simulink model "dlqr_reg_lin_model"  (R2017a)
settings: Solver=ode5  StartTime=0.0  StopTime=7  FixedStep=0.0056  RelTol=1e-3
values from neighbouring files (symbols this model uses):
  A = sys_ss.A    [dlqr_reg.m]
  B = sys_ss.B(:,1)    [dlqr_reg.m]
  C = sys_ss.C    [dlqr_reg.m]
  D = sys_ss.D(1)    [dlqr_reg.m]
undefined symbols (not defined in the file or in its folder): DiscIntNeverNeededParam, K1
libraries: cstblocks x1
settings Model: Creator=user  LastModifiedBy=user

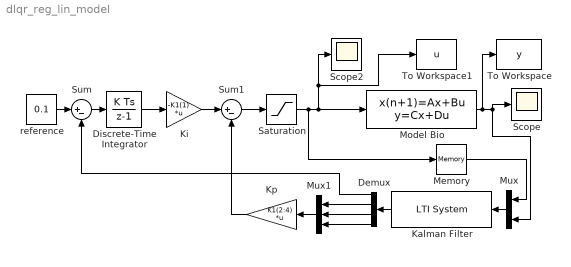
== system dlqr_reg_lin_model ==
  Demux : Demux
  Discrete-Time Integrator : DiscreteIntegrator  InitialConditionSetting=State (most efficient)  SampleTime=-1  ICPrevOutput=DiscIntNeverNeededParam  ICPrevScaledInput=DiscIntNeverNeededParam
  Kalman Filter : cstblocks/LTI System  sys=Kal  IC=[]
  Ki : Gain  Gain=-K1(1)  Multiplication=Matrix(K*u)
  Kp : Gain  Gain=K1(2:4)  Multiplication=Matrix(K*u)
  Memory : Memory
  Model Bio : DiscreteStateSpace  A=A  B=B  C=C  D=D  SampleTime=-1
  Mux : Mux  Inputs=2
  Mux1 : Mux  Inputs=3
  Saturation : Saturate  UpperLimit=1  LowerLimit=0
  Scope : Scope
  Scope2 : Scope
  Sum : Sum  Inputs=|+-
  Sum1 : Sum  Inputs=|+-
  To Workspace : ToWorkspace  VariableName=y  SaveFormat=Timeseries  SampleTime=-1
  To Workspace1 : ToWorkspace  VariableName=u  SaveFormat=Timeseries  SampleTime=-1
  "reference " : Constant  Value=0.1  SampleTime=0.0056
  wires:
  Discrete-Time Integrator/1 -> Ki/1
  "reference "/1 -> Sum/1
  Sum/1 -> Discrete-Time Integrator/1
  Ki/1 -> Sum1/1
  Sum1/1 -> Saturation/1
  Kp/1 -> Sum1/2
  Model Bio/1 -> Mux/2, Scope/1, To Workspace/1
  Mux/1 -> Kalman Filter/1
  Kalman Filter/1 -> Demux/1
  Demux/1 -> Sum/2
  Demux/2 -> Mux1/1
  Demux/3 -> Mux1/2
  Demux/4 -> Mux1/3
  Mux1/1 -> Kp/1
  Memory/1 -> Mux/1
  Saturation/1 -> Scope2/1, To Workspace1/1, Model Bio/1, Memory/1
